simulink model "thermalResistanceNetworkV3"  (R2021b)
settings: Solver=VariableStepAuto  StartTime=0.0  StopTime=numSec  RelTol=1e-3
undefined symbols (not defined in the file): A_rad, A_solararray_face, m_45bracket, m_XRD, Q_PH
libraries: fl_lib x170, nesl_utility x39
(part 1 of 2)
settings Model: Creator=home  LastModifiedBy=benmay

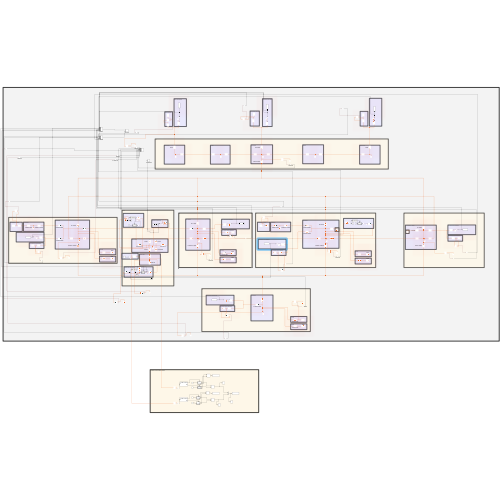
[thumbnail: Simulink's stored preview of the top-level diagram]
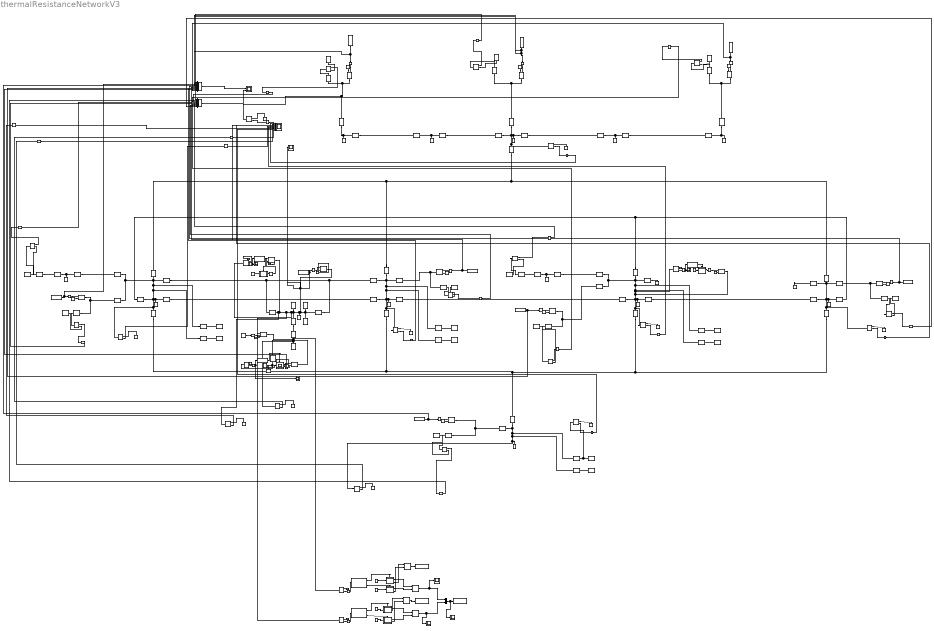
== system thermalResistanceNetworkV3 ==
  note: System
  note: Internal
  note: -X
  note: -Y
  note: Remove
  note: -Z
  note: +Y
  note: +Z Radiator to Space
  note: +Z GRD
  note: +Z XRD
  note: Battery Box
  note: Avioncs Box
  note: +Z Chassis Output Radiation
  note: +Z
  note: +Z Chassis Input Radiation
  note: +X
  note: +Z Radiator
  note: Hinge 2
  note: +X Chassis
  note: Hinge 1
  note: Solar Array 1
  note: Solar Array 2
  note: -X Chassis
  note: +Z Chassis
  note: +Y Chassis
  note: -Y Chassis (To Earth)
  note: -Z Radiator
  note: -Z Chassis
  note: -Z Chassis Output Radiation
  note: -Z Chassis Input Radiation
  note: -X Chassis Output Radiation
  note: -X Chassis Input Radiation
  note: +Y GRD
  note: +Y XRD
  note: -Z GRD
  note: -Z XRD
  note: -X GRD
  note: -X XRD
  note: +Y Chassis Output Radiation
  note: +Y Chassis Input Radiation
  note: -Z Radiator to Space
  note: Remove
  note: -Y Chassis Output Radiation
  note: -Y Chassis Input Radiation
  note: Output Rad SA1
  note: SA1 Input Radiation
  note: +X Chassis Rad Out
  note: +X Chassis Input Rad
  note: Output Rad SA2
  note: SA2 Input Radiation
  note: Battery Heat Gen.
  note: Operational Heat Gen.
  note: Avioncs Box Patch Heater
  note: -Z Patch Heater
  note: Battery Box Patch Heater
  note: PH/RA Brute Force Method Control
  +X Chassis : fl_lib/Thermal/Thermal Elements/Thermal Mass  mass=m_CHX kg  sp_heat=447 J/kg/K  T_specify=off  T_priority=High  T=300 K  T_nominal_specify=off  T_nominal_unit=K  T_nominal_value=1  Q_specify=off  Q_priority=None  Q=0 W  Q_nominal_specify=off  Q_nominal_unit=W  Q_nominal_value=1
  +X Chassis to Hinge 1 : fl_lib/Thermal/Thermal Elements/Thermal Resistance  resistance=R_chassisY K/W  T_specify=off  T_priority=None  T=0 K  T_nominal_specify=off  T_nominal_unit=K  T_nominal_value=1  Q_specify=off  Q_priority=None  Q=0 W  Q_nominal_specify=off  Q_nominal_unit=W  Q_nominal_value=1
      settings: SourceProductBaseCode=SS
  +X Chassis to Hinge 2 : fl_lib/Thermal/Thermal Elements/Thermal Resistance  resistance=R_chassisY K/W  T_specify=off  T_priority=None  T=0 K  T_nominal_specify=off  T_nominal_unit=K  T_nominal_value=1  Q_specify=off  Q_priority=None  Q=0 W  Q_nominal_specify=off  Q_nominal_unit=W  Q_nominal_value=1
      settings: SourceProductBaseCode=SS
  +X Chassis1 : fl_lib/Thermal/Thermal Elements/Thermal Mass  mass=1 kg  sp_heat=447 J/kg/K  T_specify=off  T_priority=High  T=300 K  T_nominal_specify=off  T_nominal_unit=K  T_nominal_value=1  Q_specify=off  Q_priority=None  Q=0 W  Q_nominal_specify=off  Q_nominal_unit=W  Q_nominal_value=1
  +Y Chassis : fl_lib/Thermal/Thermal Elements/Thermal Mass  mass=m_CHYZ kg  sp_heat=447 J/kg/K  T_specify=off  T_priority=High  T=300 K  T_nominal_specify=off  T_nominal_unit=K  T_nominal_value=1  Q_specify=off  Q_priority=None  Q=0 W  Q_nominal_specify=off  Q_nominal_unit=W  Q_nominal_value=1
  +Y Chassis to +Z Chassis : fl_lib/Thermal/Thermal Elements/Thermal Resistance  resistance=R_chassisXZ K/W  T_specify=off  T_priority=None  T=0 K  T_nominal_specify=off  T_nominal_unit=K  T_nominal_value=1  Q_specify=off  Q_priority=None  Q=0 W  Q_nominal_specify=off  Q_nominal_unit=W  Q_nominal_value=1
      settings: SourceProductBaseCode=SS
  +Y Chassis to -X Chassis : fl_lib/Thermal/Thermal Elements/Thermal Resistance  resistance=R_chassisXZ K/W  T_specify=off  T_priority=None  T=0 K  T_nominal_specify=off  T_nominal_unit=K  T_nominal_value=1  Q_specify=off  Q_priority=None  Q=0 W  Q_nominal_specify=off  Q_nominal_unit=W  Q_nominal_value=1
      settings: SourceProductBaseCode=SS
  +Y Chassis to -Z Chassis : fl_lib/Thermal/Thermal Elements/Thermal Resistance  resistance=R_chassisXZ K/W  T_specify=off  T_priority=None  T=0 K  T_nominal_specify=off  T_nominal_unit=K  T_nominal_value=1  Q_specify=off  Q_priority=None  Q=0 W  Q_nominal_specify=off  Q_nominal_unit=W  Q_nominal_value=1
      settings: SourceProductBaseCode=SS
  +Y Chassis to GRD : fl_lib/Thermal/Thermal Elements/Thermal Resistance  resistance=R_XRD K/W  T_specify=off  T_priority=None  T=0 K  T_nominal_specify=off  T_nominal_unit=K  T_nominal_value=1  Q_specify=off  Q_priority=None  Q=0 W  Q_nominal_specify=off  Q_nominal_unit=W  Q_nominal_value=1
      settings: SourceProductBaseCode=SS
  +Y Chassis to Inside : fl_lib/Thermal/Thermal Elements/Thermal Resistance  resistance=R_chassisXZ K/W  T_specify=off  T_priority=None  T=0 K  T_nominal_specify=off  T_nominal_unit=K  T_nominal_value=1  Q_specify=off  Q_priority=None  Q=0 W  Q_nominal_specify=off  Q_nominal_unit=W  Q_nominal_value=1
      settings: SourceProductBaseCode=SS
  +Y Chassis to Outside : fl_lib/Thermal/Thermal Elements/Thermal Resistance  resistance=R_chassisXZ K/W  T_specify=off  T_priority=None  T=0 K  T_nominal_specify=off  T_nominal_unit=K  T_nominal_value=1  Q_specify=off  Q_priority=None  Q=0 W  Q_nominal_specify=off  Q_nominal_unit=W  Q_nominal_value=1
      settings: SourceProductBaseCode=SS
  +Y Chassis to XRD : fl_lib/Thermal/Thermal Elements/Thermal Resistance  resistance=R_XRD K/W  T_specify=off  T_priority=None  T=0 K  T_nominal_specify=off  T_nominal_unit=K  T_nominal_value=1  Q_specify=off  Q_priority=None  Q=0 W  Q_nominal_specify=off  Q_nominal_unit=W  Q_nominal_value=1
      settings: SourceProductBaseCode=SS
  +Y GRD : fl_lib/Thermal/Thermal Elements/Thermal Mass  mass=m_GRD kg  sp_heat=447 J/kg/K  T_specify=off  T_priority=High  T=300 K  T_nominal_specify=off  T_nominal_unit=K  T_nominal_value=1  Q_specify=off  Q_priority=None  Q=0 W  Q_nominal_specify=off  Q_nominal_unit=W  Q_nominal_value=1
  +Y XRD : fl_lib/Thermal/Thermal Elements/Thermal Mass  mass=1.5*m_XRD + 0.5*m_45bracket kg  sp_heat=447 J/kg/K  T_specify=off  T_priority=High  T=300 K  T_nominal_specify=off  T_nominal_unit=K  T_nominal_value=1  Q_specify=off  Q_priority=None  Q=0 W  Q_nominal_specify=off  Q_nominal_unit=W  Q_nominal_value=1
  +Z Chassis : fl_lib/Thermal/Thermal Elements/Thermal Mass  mass=m_CHYZ kg  sp_heat=447 J/kg/K  T_specify=off  T_priority=High  T=300 K  T_nominal_specify=off  T_nominal_unit=K  T_nominal_value=1  Q_specify=off  Q_priority=None  Q=0 W  Q_nominal_specify=off  Q_nominal_unit=W  Q_nominal_value=1
  +Z Chassis to +Y Chassis : fl_lib/Thermal/Thermal Elements/Thermal Resistance  resistance=R_chassisXZ K/W  T_specify=off  T_priority=None  T=0 K  T_nominal_specify=off  T_nominal_unit=K  T_nominal_value=1  Q_specify=off  Q_priority=None  Q=0 W  Q_nominal_specify=off  Q_nominal_unit=W  Q_nominal_value=1
      settings: SourceProductBaseCode=SS
  +Z Chassis to -X Chassis : fl_lib/Thermal/Thermal Elements/Thermal Resistance  resistance=R_chassisXZ K/W  T_specify=off  T_priority=None  T=0 K  T_nominal_specify=off  T_nominal_unit=K  T_nominal_value=1  Q_specify=off  Q_priority=None  Q=0 W  Q_nominal_specify=off  Q_nominal_unit=W  Q_nominal_value=1
      settings: SourceProductBaseCode=SS
  +Z Chassis to -Y Chassis : fl_lib/Thermal/Thermal Elements/Thermal Resistance  resistance=R_chassisXZ K/W  T_specify=off  T_priority=None  T=0 K  T_nominal_specify=off  T_nominal_unit=K  T_nominal_value=1  Q_specify=off  Q_priority=None  Q=0 W  Q_nominal_specify=off  Q_nominal_unit=W  Q_nominal_value=1
      settings: SourceProductBaseCode=SS
  +Z Chassis to GRD : fl_lib/Thermal/Thermal Elements/Thermal Resistance  resistance=R_XRD K/W  T_specify=off  T_priority=None  T=0 K  T_nominal_specify=off  T_nominal_unit=K  T_nominal_value=1  Q_specify=off  Q_priority=None  Q=0 W  Q_nominal_specify=off  Q_nominal_unit=W  Q_nominal_value=1
      settings: SourceProductBaseCode=SS
  +Z Chassis to Inside : fl_lib/Thermal/Thermal Elements/Thermal Resistance  resistance=R_chassisXZ K/W  T_specify=off  T_priority=None  T=0 K  T_nominal_specify=off  T_nominal_unit=K  T_nominal_value=1  Q_specify=off  Q_priority=None  Q=0 W  Q_nominal_specify=off  Q_nominal_unit=W  Q_nominal_value=1
      settings: SourceProductBaseCode=SS
  +Z Chassis to Outside : fl_lib/Thermal/Thermal Elements/Thermal Resistance  resistance=R_chassisXZ K/W  T_specify=off  T_priority=None  T=0 K  T_nominal_specify=off  T_nominal_unit=K  T_nominal_value=1  Q_specify=off  Q_priority=None  Q=0 W  Q_nominal_specify=off  Q_nominal_unit=W  Q_nominal_value=1
      settings: SourceProductBaseCode=SS
  +Z Chassis to Radiator : fl_lib/Thermal/Thermal Elements/Thermal Resistance  resistance=R_chassisXZ K/W  T_specify=off  T_priority=None  T=0 K  T_nominal_specify=off  T_nominal_unit=K  T_nominal_value=1  Q_specify=off  Q_priority=None  Q=0 W  Q_nominal_specify=off  Q_nominal_unit=W  Q_nominal_value=1
      settings: SourceProductBaseCode=SS
  +Z Chassis to XRD : fl_lib/Thermal/Thermal Elements/Thermal Resistance  resistance=R_XRD K/W  T_specify=off  T_priority=None  T=0 K  T_nominal_specify=off  T_nominal_unit=K  T_nominal_value=1  Q_specify=off  Q_priority=None  Q=0 W  Q_nominal_specify=off  Q_nominal_unit=W  Q_nominal_value=1
      settings: SourceProductBaseCode=SS
  +Z GRD : fl_lib/Thermal/Thermal Elements/Thermal Mass  mass=m_GRD kg  sp_heat=447 J/kg/K  T_specify=off  T_priority=High  T=300 K  T_nominal_specify=off  T_nominal_unit=K  T_nominal_value=1  Q_specify=off  Q_priority=None  Q=0 W  Q_nominal_specify=off  Q_nominal_unit=W  Q_nominal_value=1
  +Z Radiator : fl_lib/Thermal/Thermal Elements/Thermal Mass  mass=m_radiator kg  sp_heat=447 J/kg/K  T_specify=off  T_priority=High  T=300 K  T_nominal_specify=off  T_nominal_unit=K  T_nominal_value=1  Q_specify=off  Q_priority=None  Q=0 W  Q_nominal_specify=off  Q_nominal_unit=W  Q_nominal_value=1
  +Z Radiator to +Z Chassis : fl_lib/Thermal/Thermal Elements/Thermal Resistance  resistance=R_rad_chassis_top K/W  T_specify=off  T_priority=None  T=0 K  T_nominal_specify=off  T_nominal_unit=K  T_nominal_value=1  Q_specify=off  Q_priority=None  Q=0 W  Q_nominal_specify=off  Q_nominal_unit=W  Q_nominal_value=1
      settings: SourceProductBaseCode=SS
  +Z Radiator to Space : fl_lib/Thermal/Thermal Elements/Thermal Resistance  resistance=R_rad_chassis_top K/W  T_specify=off  T_priority=None  T=0 K  T_nominal_specify=off  T_nominal_unit=K  T_nominal_value=1  Q_specify=off  Q_priority=None  Q=0 W  Q_nominal_specify=off  Q_nominal_unit=W  Q_nominal_value=1
      settings: SourceProductBaseCode=SS
  +Z XRD : fl_lib/Thermal/Thermal Elements/Thermal Mass  mass=m_XRD kg  sp_heat=447 J/kg/K  T_specify=off  T_priority=High  T=300 K  T_nominal_specify=off  T_nominal_unit=K  T_nominal_value=1  Q_specify=off  Q_priority=None  Q=0 W  Q_nominal_specify=off  Q_nominal_unit=W  Q_nominal_value=1
  -X Chassis to GRD : fl_lib/Thermal/Thermal Elements/Thermal Resistance  resistance=R_XRD K/W  T_specify=off  T_priority=None  T=0 K  T_nominal_specify=off  T_nominal_unit=K  T_nominal_value=1  Q_specify=off  Q_priority=None  Q=0 W  Q_nominal_specify=off  Q_nominal_unit=W  Q_nominal_value=1
      settings: SourceProductBaseCode=SS
  -X Chassis to Outside : fl_lib/Thermal/Thermal Elements/Thermal Resistance  resistance=R_chassisY K/W  T_specify=off  T_priority=None  T=0 K  T_nominal_specify=off  T_nominal_unit=K  T_nominal_value=1  Q_specify=off  Q_priority=None  Q=0 W  Q_nominal_specify=off  Q_nominal_unit=W  Q_nominal_value=1
      settings: SourceProductBaseCode=SS
  -X Chassis to XRD : fl_lib/Thermal/Thermal Elements/Thermal Resistance  resistance=R_XRD K/W  T_specify=off  T_priority=None  T=0 K  T_nominal_specify=off  T_nominal_unit=K  T_nominal_value=1  Q_specify=off  Q_priority=None  Q=0 W  Q_nominal_specify=off  Q_nominal_unit=W  Q_nominal_value=1
      settings: SourceProductBaseCode=SS
  -X GRD : fl_lib/Thermal/Thermal Elements/Thermal Mass  mass=m_GRD kg  sp_heat=447 J/kg/K  T_specify=off  T_priority=High  T=300 K  T_nominal_specify=off  T_nominal_unit=K  T_nominal_value=1  Q_specify=off  Q_priority=None  Q=0 W  Q_nominal_specify=off  Q_nominal_unit=W  Q_nominal_value=1
  -X XRD : fl_lib/Thermal/Thermal Elements/Thermal Mass  mass=1.5*m_XRD + 0.5*m_45bracket kg  sp_heat=447 J/kg/K  T_specify=off  T_priority=High  T=300 K  T_nominal_specify=off  T_nominal_unit=K  T_nominal_value=1  Q_specify=off  Q_priority=None  Q=0 W  Q_nominal_specify=off  Q_nominal_unit=W  Q_nominal_value=1
  -Y Chassis : fl_lib/Thermal/Thermal Elements/Thermal Mass  mass=m_CHYZ kg  sp_heat=447 J/kg/K  T_specify=off  T_priority=High  T=300 K  T_nominal_specify=off  T_nominal_unit=K  T_nominal_value=1  Q_specify=off  Q_priority=None  Q=0 W  Q_nominal_specify=off  Q_nominal_unit=W  Q_nominal_value=1
  -Y Chassis to +Z Chassis : fl_lib/Thermal/Thermal Elements/Thermal Resistance  resistance=R_chassisXZ K/W  T_specify=off  T_priority=None  T=0 K  T_nominal_specify=off  T_nominal_unit=K  T_nominal_value=1  Q_specify=off  Q_priority=None  Q=0 W  Q_nominal_specify=off  Q_nominal_unit=W  Q_nominal_value=1
      settings: SourceProductBaseCode=SS
  -Y Chassis to -Z Chassis : fl_lib/Thermal/Thermal Elements/Thermal Resistance  resistance=R_chassisXZ K/W  T_specify=off  T_priority=None  T=0 K  T_nominal_specify=off  T_nominal_unit=K  T_nominal_value=1  Q_specify=off  Q_priority=None  Q=0 W  Q_nominal_specify=off  Q_nominal_unit=W  Q_nominal_value=1
      settings: SourceProductBaseCode=SS
  -Y to Inside : fl_lib/Thermal/Thermal Elements/Thermal Resistance  resistance=R_chassisXZ K/W  T_specify=off  T_priority=None  T=0 K  T_nominal_specify=off  T_nominal_unit=K  T_nominal_value=1  Q_specify=off  Q_priority=None  Q=0 W  Q_nominal_specify=off  Q_nominal_unit=W  Q_nominal_value=1
      settings: SourceProductBaseCode=SS
  -Y to Outside : fl_lib/Thermal/Thermal Elements/Thermal Resistance  resistance=R_chassisXZ K/W  T_specify=off  T_priority=None  T=0 K  T_nominal_specify=off  T_nominal_unit=K  T_nominal_value=1  Q_specify=off  Q_priority=None  Q=0 W  Q_nominal_specify=off  Q_nominal_unit=W  Q_nominal_value=1
      settings: SourceProductBaseCode=SS
  -Z Chassis : fl_lib/Thermal/Thermal Elements/Thermal Mass  mass=m_CHYZ kg  sp_heat=447 J/kg/K  T_specify=off  T_priority=High  T=300 K  T_nominal_specify=off  T_nominal_unit=K  T_nominal_value=1  Q_specify=off  Q_priority=None  Q=0 W  Q_nominal_specify=off  Q_nominal_unit=W  Q_nominal_value=1
  -Z Chassis to +Y Chassis : fl_lib/Thermal/Thermal Elements/Thermal Resistance  resistance=R_chassisXZ K/W  T_specify=off  T_priority=None  T=0 K  T_nominal_specify=off  T_nominal_unit=K  T_nominal_value=1  Q_specify=off  Q_priority=None  Q=0 W  Q_nominal_specify=off  Q_nominal_unit=W  Q_nominal_value=1
      settings: SourceProductBaseCode=SS
  -Z Chassis to -X Chassis1 : fl_lib/Thermal/Thermal Elements/Thermal Resistance  resistance=R_chassisXZ K/W  T_specify=off  T_priority=None  T=0 K  T_nominal_specify=off  T_nominal_unit=K  T_nominal_value=1  Q_specify=off  Q_priority=None  Q=0 W  Q_nominal_specify=off  Q_nominal_unit=W  Q_nominal_value=1
      settings: SourceProductBaseCode=SS
  -Z Chassis to -Y Chassis : fl_lib/Thermal/Thermal Elements/Thermal Resistance  resistance=R_chassisXZ K/W  T_specify=off  T_priority=None  T=0 K  T_nominal_specify=off  T_nominal_unit=K  T_nominal_value=1  Q_specify=off  Q_priority=None  Q=0 W  Q_nominal_specify=off  Q_nominal_unit=W  Q_nominal_value=1
      settings: SourceProductBaseCode=SS
  -Z Chassis to GRD : fl_lib/Thermal/Thermal Elements/Thermal Resistance  resistance=R_XRD K/W  T_specify=off  T_priority=None  T=0 K  T_nominal_specify=off  T_nominal_unit=K  T_nominal_value=1  Q_specify=off  Q_priority=None  Q=0 W  Q_nominal_specify=off  Q_nominal_unit=W  Q_nominal_value=1
      settings: SourceProductBaseCode=SS
  -Z Chassis to Inside : fl_lib/Thermal/Thermal Elements/Thermal Resistance  resistance=1 K/W  T_specify=off  T_priority=None  T=0 K  T_nominal_specify=off  T_nominal_unit=K  T_nominal_value=1  Q_specify=off  Q_priority=None  Q=0 W  Q_nominal_specify=off  Q_nominal_unit=W  Q_nominal_value=1
      settings: SourceProductBaseCode=SS
  -Z Chassis to Outside : fl_lib/Thermal/Thermal Elements/Thermal Resistance  resistance=R_chassisXZ K/W  T_specify=off  T_priority=None  T=0 K  T_nominal_specify=off  T_nominal_unit=K  T_nominal_value=1  Q_specify=off  Q_priority=None  Q=0 W  Q_nominal_specify=off  Q_nominal_unit=W  Q_nominal_value=1
      settings: SourceProductBaseCode=SS
  -Z Chassis to Radiator : fl_lib/Thermal/Thermal Elements/Thermal Resistance  resistance=R_chassisXZ K/W  T_specify=off  T_priority=None  T=0 K  T_nominal_specify=off  T_nominal_unit=K  T_nominal_value=1  Q_specify=off  Q_priority=None  Q=0 W  Q_nominal_specify=off  Q_nominal_unit=W  Q_nominal_value=1
      settings: SourceProductBaseCode=SS
  -Z Chassis to XRD : fl_lib/Thermal/Thermal Elements/Thermal Resistance  resistance=R_XRD K/W  T_specify=off  T_priority=None  T=0 K  T_nominal_specify=off  T_nominal_unit=K  T_nominal_value=1  Q_specify=off  Q_priority=None  Q=0 W  Q_nominal_specify=off  Q_nominal_unit=W  Q_nominal_value=1
      settings: SourceProductBaseCode=SS
  -Z GRD : fl_lib/Thermal/Thermal Elements/Thermal Mass  mass=m_GRD kg  sp_heat=447 J/kg/K  T_specify=off  T_priority=High  T=300 K  T_nominal_specify=off  T_nominal_unit=K  T_nominal_value=1  Q_specify=off  Q_priority=None  Q=0 W  Q_nominal_specify=off  Q_nominal_unit=W  Q_nominal_value=1
  -Z Radiator : fl_lib/Thermal/Thermal Elements/Thermal Mass  mass=m_radiator kg  sp_heat=447 J/kg/K  T_specify=off  T_priority=High  T=300 K  T_nominal_specify=off  T_nominal_unit=K  T_nominal_value=1  Q_specify=off  Q_priority=None  Q=0 W  Q_nominal_specify=off  Q_nominal_unit=W  Q_nominal_value=1
  -Z Radiator to -Z Chassis : fl_lib/Thermal/Thermal Elements/Thermal Resistance  resistance=R_chassisXZ K/W  T_specify=off  T_priority=None  T=0 K  T_nominal_specify=off  T_nominal_unit=K  T_nominal_value=1  Q_specify=off  Q_priority=None  Q=0 W  Q_nominal_specify=off  Q_nominal_unit=W  Q_nominal_value=1
      settings: SourceProductBaseCode=SS
  -Z Radiator to Space : fl_lib/Thermal/Thermal Elements/Thermal Resistance  resistance=R_chassisXZ K/W  T_specify=off  T_priority=None  T=0 K  T_nominal_specify=off  T_nominal_unit=K  T_nominal_value=1  Q_specify=off  Q_priority=None  Q=0 W  Q_nominal_specify=off  Q_nominal_unit=W  Q_nominal_value=1
      settings: SourceProductBaseCode=SS
  -Z XRD : fl_lib/Thermal/Thermal Elements/Thermal Mass  mass=2*m_XRD + 0.5*m_45bracket kg  sp_heat=447 J/kg/K  T_specify=off  T_priority=High  T=300 K  T_nominal_specify=off  T_nominal_unit=K  T_nominal_value=1  Q_specify=off  Q_priority=None  Q=0 W  Q_nominal_specify=off  Q_nominal_unit=W  Q_nominal_value=1
  Avionics -Y : fl_lib/Thermal/Thermal Elements/Thermal Resistance  resistance=R_AB_internal K/W  T_specify=off  T_priority=None  T=0 K  T_nominal_specify=off  T_nominal_unit=K  T_nominal_value=1  Q_specify=off  Q_priority=None  Q=0 W  Q_nominal_specify=off  Q_nominal_unit=W  Q_nominal_value=1
      settings: SourceProductBaseCode=SS
  Avionics -Z : fl_lib/Thermal/Thermal Elements/Thermal Resistance  resistance=1 K/W  T_specify=off  T_priority=None  T=0 K  T_nominal_specify=off  T_nominal_unit=K  T_nominal_value=1  Q_specify=off  Q_priority=None  Q=0 W  Q_nominal_specify=off  Q_nominal_unit=W  Q_nominal_value=1
      settings: SourceProductBaseCode=SS
  Avionics Bottom : fl_lib/Thermal/Thermal Elements/Thermal Resistance  resistance=1 K/W  T_specify=off  T_priority=None  T=0 K  T_nominal_specify=off  T_nominal_unit=K  T_nominal_value=1  Q_specify=off  Q_priority=None  Q=0 W  Q_nominal_specify=off  Q_nominal_unit=W  Q_nominal_value=1
      settings: SourceProductBaseCode=SS
  Avionics Box : fl_lib/Thermal/Thermal Elements/Thermal Mass  mass=m_AB kg  sp_heat=447 J/kg/K  T_specify=on  T_priority=High  T=282 K  T_nominal_specify=off  T_nominal_unit=K  T_nominal_value=1  Q_specify=off  Q_priority=None  Q=0 W  Q_nominal_specify=off  Q_nominal_unit=W  Q_nominal_value=1
  Avionics Box to +Y : fl_lib/Thermal/Thermal Elements/Thermal Resistance  resistance=R_AB_internal K/W  T_specify=off  T_priority=None  T=0 K  T_nominal_specify=off  T_nominal_unit=K  T_nominal_value=1  Q_specify=off  Q_priority=None  Q=0 W  Q_nominal_specify=off  Q_nominal_unit=W  Q_nominal_value=1
      settings: SourceProductBaseCode=SS
  Avionics Box to +Z : fl_lib/Thermal/Thermal Elements/Thermal Resistance  resistance=R_AB_internal K/W  T_specify=off  T_priority=None  T=0 K  T_nominal_specify=off  T_nominal_unit=K  T_nominal_value=1  Q_specify=off  Q_priority=None  Q=0 W  Q_nominal_specify=off  Q_nominal_unit=W  Q_nominal_value=1
      settings: SourceProductBaseCode=SS
  Avionics Top : fl_lib/Thermal/Thermal Elements/Thermal Resistance  resistance=1 K/W  T_specify=off  T_priority=None  T=0 K  T_nominal_specify=off  T_nominal_unit=K  T_nominal_value=1  Q_specify=off  Q_priority=None  Q=0 W  Q_nominal_specify=off  Q_nominal_unit=W  Q_nominal_value=1
      settings: SourceProductBaseCode=SS
  AvionicsBox : nesl_utility/PS-Simulink Converter  PhysicalDomain=network_engine_domain  SubClassName=ps_output  LeftPortType=input  RightPortType=output  PseudoPeriodic=off  Frequencies=[]  Unit=K  AffineConversion=off
      settings: SourceProductBaseCode=PW,SS
  Battery Box : fl_lib/Thermal/Thermal Elements/Thermal Mass  mass=m_BB kg  sp_heat=447 J/kg/K  T_specify=on  T_priority=High  T=282 K  T_nominal_specify=off  T_nominal_unit=K  T_nominal_value=1  Q_specify=off  Q_priority=None  Q=0 W  Q_nominal_specify=off  Q_nominal_unit=W  Q_nominal_value=1
  Battery Box to Avionics : fl_lib/Thermal/Thermal Elements/Thermal Resistance  resistance=R_BB_internal K/W  T_specify=off  T_priority=None  T=0 K  T_nominal_specify=off  T_nominal_unit=K  T_nominal_value=1  Q_specify=off  Q_priority=None  Q=0 W  Q_nominal_specify=off  Q_nominal_unit=W  Q_nominal_value=1
      settings: SourceProductBaseCode=SS
  BatteryBox : nesl_utility/PS-Simulink Converter  PhysicalDomain=network_engine_domain  SubClassName=ps_output  LeftPortType=input  RightPortType=output  PseudoPeriodic=off  Frequencies=[]  Unit=K  AffineConversion=off
      settings: SourceProductBaseCode=PW,SS
  "Bottom +X Chassis " : fl_lib/Thermal/Thermal Elements/Thermal Resistance  resistance=R_chassisY K/W  T_specify=off  T_priority=None  T=0 K  T_nominal_specify=off  T_nominal_unit=K  T_nominal_value=1  Q_specify=off  Q_priority=None  Q=0 W  Q_nominal_specify=off  Q_nominal_unit=W  Q_nominal_value=1
      settings: SourceProductBaseCode=SS
  "Bottom -Y Chassis " : fl_lib/Thermal/Thermal Elements/Thermal Resistance  resistance=R_chassisXZ K/W  T_specify=off  T_priority=None  T=0 K  T_nominal_specify=off  T_nominal_unit=K  T_nominal_value=1  Q_specify=off  Q_priority=None  Q=0 W  Q_nominal_specify=off  Q_nominal_unit=W  Q_nominal_value=1
      settings: SourceProductBaseCode=SS
  Constant : Constant  Value=0.9
  Constant1 : Constant  Value=0
  Constant2 : Constant  Value=Q_PH/3
  Constant3 : Constant  Value=0
  Constant4 : Constant
  Constant5 : Constant
  Constant6 : Constant  Value=Q_PH/3
  Constant7 : Constant  Value=Q_PH/3
  Controlled Heat Flow Rate Source{,1..12} (13 alike) : fl_lib/Thermal/Thermal Sources/Controlled Heat Flow Rate Source
  From Workspace1 : FromWorkspace  VariableName=Q_SA_TS  SampleTime=300
  From Workspace10 : FromWorkspace  VariableName=Q_Gen_TS  SampleTime=300
  From Workspace2 : FromWorkspace  VariableName=Q_Xpos_TS  SampleTime=300
  From Workspace3 : FromWorkspace  VariableName=Q_SA_TS  SampleTime=300
  From Workspace4 : FromWorkspace  VariableName=Q_Zpos_TS  SampleTime=300
  From Workspace5 : FromWorkspace  VariableName=Q_Ypos_TS  SampleTime=300
  From Workspace6 : FromWorkspace  VariableName=Q_Zneg_TS  SampleTime=300
  From Workspace7 : FromWorkspace  VariableName=Q_Xneg_TS  SampleTime=300
  From Workspace8 : FromWorkspace  VariableName=Q_Yneg_TS  SampleTime=300
  Heat Flow Rate Sensor{1..10} (10 alike) : fl_lib/Thermal/Thermal Sensors/Heat Flow Rate Sensor
      settings: SourceProductBaseCode=SS
  Heat In : Sum  Inputs=+++++++++++
  Heat Out : Sum  Inputs=++++++++++
  Heat in/out : Scope  NumInputPorts=2
  Hinge 1 : fl_lib/Thermal/Thermal Elements/Thermal Mass  mass=m_hinge kg  sp_heat=887 J/kg/K  T_specify=off  T_priority=High  T=300 K  T_nominal_specify=off  T_nominal_unit=K  T_nominal_value=1  Q_specify=off  Q_priority=None  Q=0 W  Q_nominal_specify=off  Q_nominal_unit=W  Q_nominal_value=1
  Hinge 1 to +X Chassis : fl_lib/Thermal/Thermal Elements/Thermal Resistance  resistance=R_Hinge K/W  T_specify=off  T_priority=None  T=0 K  T_nominal_specify=off  T_nominal_unit=K  T_nominal_value=1  Q_specify=off  Q_priority=None  Q=0 W  Q_nominal_specify=off  Q_nominal_unit=W  Q_nominal_value=1
      settings: SourceProductBaseCode=SS
  Hinge 1 to SA1 : fl_lib/Thermal/Thermal Elements/Thermal Resistance  resistance=R_Hinge K/W  T_specify=off  T_priority=None  T=0 K  T_nominal_specify=off  T_nominal_unit=K  T_nominal_value=1  Q_specify=off  Q_priority=None  Q=0 W  Q_nominal_specify=off  Q_nominal_unit=W  Q_nominal_value=1
      settings: SourceProductBaseCode=SS
  Hinge 2 : fl_lib/Thermal/Thermal Elements/Thermal Mass  mass=m_hinge kg  sp_heat=447 J/kg/K  T_specify=off  T_priority=High  T=300 K  T_nominal_specify=off  T_nominal_unit=K  T_nominal_value=1  Q_specify=off  Q_priority=None  Q=0 W  Q_nominal_specify=off  Q_nominal_unit=W  Q_nominal_value=1
  Hinge 2 to +X Chassis : fl_lib/Thermal/Thermal Elements/Thermal Resistance  resistance=R_Hinge K/W  T_specify=off  T_priority=None  T=0 K  T_nominal_specify=off  T_nominal_unit=K  T_nominal_value=1  Q_specify=off  Q_priority=None  Q=0 W  Q_nominal_specify=off  Q_nominal_unit=W  Q_nominal_value=1
      settings: SourceProductBaseCode=SS
  Hinge 2 to SA2 : fl_lib/Thermal/Thermal Elements/Thermal Resistance  resistance=R_Hinge K/W  T_specify=off  T_priority=None  T=0 K  T_nominal_specify=off  T_nominal_unit=K  T_nominal_value=1  Q_specify=off  Q_priority=None  Q=0 W  Q_nominal_specify=off  Q_nominal_unit=W  Q_nominal_value=1
      settings: SourceProductBaseCode=SS
  If Action Subsystem1 : Subsystem  TreatAsAtomicUnit=on
  If Action Subsystem2 : Subsystem  TreatAsAtomicUnit=on
  If Action Subsystem3 : Subsystem  TreatAsAtomicUnit=on
  If Action Subsystem4 : Subsystem  TreatAsAtomicUnit=on
  If Action Subsystem5 : Subsystem  TreatAsAtomicUnit=on
  If Action Subsystem6 : Subsystem  TreatAsAtomicUnit=on
  If Action Subsystem7 : Subsystem  TreatAsAtomicUnit=on
  If1 : If  IfExpression=u1 > 288.5 | u1<278.15
  If2 : If  IfExpression=u1 < 283.15  ShowElse=off
  If3 : If  IfExpression=u1 < 273.15  ShowElse=off
  If4 : If  IfExpression=u1 > 308.5 | u1<278.15
  If5 : If  IfExpression=u1 < 288.15  ShowElse=off
  Inside Edge SA1 : fl_lib/Thermal/Thermal Elements/Thermal Resistance  resistance=R_SolarArray K/W  T_specify=off  T_priority=None  T=0 K  T_nominal_specify=off  T_nominal_unit=K  T_nominal_value=1  Q_specify=off  Q_priority=None  Q=0 W  Q_nominal_specify=off  Q_nominal_unit=W  Q_nominal_value=1
      settings: SourceProductBaseCode=SS
  Merge{,1..3} (4 alike) : Merge
  Mux : Mux  Inputs=2
  Outside Edge SA2 : fl_lib/Thermal/Thermal Elements/Thermal Resistance  resistance=R_SolarArray K/W  T_specify=off  T_priority=None  T=0 K  T_nominal_specify=off  T_nominal_unit=K  T_nominal_value=1  Q_specify=off  Q_priority=None  Q=0 W  Q_nominal_specify=off  Q_nominal_unit=W  Q_nominal_value=1
      settings: SourceProductBaseCode=SS
  PS-Simulink Converter{1..15} (15 alike) : nesl_utility/PS-Simulink Converter  PhysicalDomain=network_engine_domain  SubClassName=ps_output  LeftPortType=input  RightPortType=output  PseudoPeriodic=off  Frequencies=[]  Unit=inherit  AffineConversion=off
      settings: SourceProductBaseCode=PW,SS
  Perfect Insulator : fl_lib/Thermal/Thermal Elements/Perfect Insulator  T_specify=off  T_priority=None  T=0 K  T_nominal_specify=off  T_nominal_unit=K  T_nominal_value=1
  Perfect Insulator1 : fl_lib/Thermal/Thermal Elements/Perfect Insulator  T_specify=off  T_priority=None  T=0 K  T_nominal_specify=off  T_nominal_unit=K  T_nominal_value=1
  Power Generated : Scope
  Radiative Heat Transfer{,1,4,6} (4 alike) : fl_lib/Thermal/Thermal Elements/Radiative Heat Transfer  area=A_sidechassis m^2  rad_tr_coeff=RC_Al W/(m^2*K^4)  T_specify=off  T_priority=None  T=0 K  T_nominal_specify=off  T_nominal_unit=K  T_nominal_value=1  Q_specify=off  Q_priority=None  Q=0 W  Q_nominal_specify=off  Q_nominal_unit=W  Q_nominal_value=1
      settings: SourceProductBaseCode=SS  InternalSimscapePortConfiguration="{\"Bottom\":[],\"Left\":[{\"id\":\"A\",\"label\":\"A\",\"type\":\"foundation.thermal.thermal\"}],\"Right\":[{\"id\":\"B\",\"label\":\"B\",\"type\":\"foundation.thermal.thermal\"}],\"Top\":[]}"
  Radiative Heat Transfer2 : fl_lib/Thermal/Thermal Elements/Radiative Heat Transfer  area=A_topchassis m^2  rad_tr_coeff=RC_Al W/(m^2*K^4)  T_specify=off  T_priority=None  T=0 K  T_nominal_specify=off  T_nominal_unit=K  T_nominal_value=1  Q_specify=off  Q_priority=None  Q=0 W  Q_nominal_specify=off  Q_nominal_unit=W  Q_nominal_value=1
      settings: SourceProductBaseCode=SS  InternalSimscapePortConfiguration="{\"Bottom\":[],\"Left\":[{\"id\":\"A\",\"label\":\"A\",\"type\":\"foundation.thermal.thermal\"}],\"Right\":[{\"id\":\"B\",\"label\":\"B\",\"type\":\"foundation.thermal.thermal\"}],\"Top\":[]}"
  Radiative Heat Transfer3 : fl_lib/Thermal/Thermal Elements/Radiative Heat Transfer  area=A_rad/2 m^2  rad_tr_coeff=RC_Rad W/(m^2*K^4)  T_specify=off  T_priority=None  T=0 K  T_nominal_specify=off  T_nominal_unit=K  T_nominal_value=1  Q_specify=off  Q_priority=None  Q=0 W  Q_nominal_specify=off  Q_nominal_unit=W  Q_nominal_value=1
      settings: SourceProductBaseCode=SS  InternalSimscapePortConfiguration="{\"Bottom\":[],\"Left\":[{\"id\":\"A\",\"label\":\"A\",\"type\":\"foundation.thermal.thermal\"}],\"Right\":[{\"id\":\"B\",\"label\":\"B\",\"type\":\"foundation.thermal.thermal\"}],\"Top\":[]}"
  Radiative Heat Transfer5 : fl_lib/Thermal/Thermal Elements/Radiative Heat Transfer  area=A_rad/2 m^2  rad_tr_coeff=RC_Rad W/(m^2*K^4)  T_specify=off  T_priority=None  T=0 K  T_nominal_specify=off  T_nominal_unit=K  T_nominal_value=1  Q_specify=off  Q_priority=None  Q=0 W  Q_nominal_specify=off  Q_nominal_unit=W  Q_nominal_value=1
      settings: SourceProductBaseCode=SS  InternalSimscapePortConfiguration="{\"Bottom\":[],\"Left\":[{\"id\":\"A\",\"label\":\"A\",\"type\":\"foundation.thermal.thermal\"}],\"Right\":[{\"id\":\"B\",\"label\":\"B\",\"type\":\"foundation.thermal.thermal\"}],\"Top\":[]}"
  Radiative Heat Transfer7 : fl_lib/Thermal/Thermal Elements/Radiative Heat Transfer  area=2*A_solararray_face m^2  rad_tr_coeff=RC_SA W/(m^2*K^4)  T_specify=off  T_priority=None  T=0 K  T_nominal_specify=off  T_nominal_unit=K  T_nominal_value=1  Q_specify=off  Q_priority=None  Q=0 W  Q_nominal_specify=off  Q_nominal_unit=W  Q_nominal_value=1
      settings: SourceProductBaseCode=SS  InternalSimscapePortConfiguration="{\"Bottom\":[],\"Left\":[{\"id\":\"A\",\"label\":\"A\",\"type\":\"foundation.thermal.thermal\"}],\"Right\":[{\"id\":\"B\",\"label\":\"B\",\"type\":\"foundation.thermal.thermal\"}],\"Top\":[]}"
  Radiative Heat Transfer8 : fl_lib/Thermal/Thermal Elements/Radiative Heat Transfer  area=A_topchassis m^2  rad_tr_coeff=RC_Al W/(m^2*K^4)  T_specify=off  T_priority=None  T=0 K  T_nominal_specify=off  T_nominal_unit=K  T_nominal_value=1  Q_specify=off  Q_priority=None  Q=0 W  Q_nominal_specify=off  Q_nominal_unit=W  Q_nominal_value=1
      settings: SourceProductBaseCode=SS  InternalSimscapePortConfiguration="{\"Bottom\":[],\"Left\":[{\"id\":\"A\",\"label\":\"A\",\"type\":\"foundation.thermal.thermal\"}],\"Right\":[{\"id\":\"B\",\"label\":\"B\",\"type\":\"foundation.thermal.thermal\"}],\"Top\":[]}"
  Radiative Heat Transfer9 : fl_lib/Thermal/Thermal Elements/Radiative Heat Transfer  area=2*A_solararray_face m^2  rad_tr_coeff=RC_SA W/(m^2*K^4)  T_specify=off  T_priority=None  T=0 K  T_nominal_specify=off  T_nominal_unit=K  T_nominal_value=1  Q_specify=off  Q_priority=None  Q=0 W  Q_nominal_specify=off  Q_nominal_unit=W  Q_nominal_value=1
      settings: SourceProductBaseCode=SS  InternalSimscapePortConfiguration="{\"Bottom\":[],\"Left\":[{\"id\":\"A\",\"label\":\"A\",\"type\":\"foundation.thermal.thermal\"}],\"Right\":[{\"id\":\"B\",\"label\":\"B\",\"type\":\"foundation.thermal.thermal\"}],\"Top\":[]}"
  SA1 : fl_lib/Thermal/Thermal Elements/Thermal Mass  mass=m_SA kg  sp_heat=887 J/kg/K  T_specify=off  T_priority=High  T=300 K  T_nominal_specify=off  T_nominal_unit=K  T_nominal_value=1  Q_specify=off  Q_priority=None  Q=0 W  Q_nominal_specify=off  Q_nominal_unit=W  Q_nominal_value=1
  SA2 : fl_lib/Thermal/Thermal Elements/Thermal Mass  mass=m_SA kg  sp_heat=887 J/kg/K  T_specify=off  T_priority=High  T=300 K  T_nominal_specify=off  T_nominal_unit=K  T_nominal_value=1  Q_specify=off  Q_priority=None  Q=0 W  Q_nominal_specify=off  Q_nominal_unit=W  Q_nominal_value=1
  Scope{,1..5} (6 alike) : Scope
  Simulink-PS Converter{,1..12} (13 alike) : nesl_utility/Simulink-PS Converter  PhysicalDomain=network_engine_domain  SubClassName=ps_input  LeftPortType=input  RightPortType=output  PseudoPeriodic=off  Frequencies=[]  NoiseDistribution=none  NoiseParameters=[]  Unit=1  AffineConversion=off  FilteringAndDerivatives=provide  SimscapeFilterOrder=1  InputFilterTimeConstant=0.001  UdotUserProvided=0
      settings: SourceProductBaseCode=PW,SS
  Solar Array : nesl_utility/PS-Simulink Converter  PhysicalDomain=network_engine_domain  SubClassName=ps_output  LeftPortType=input  RightPortType=output  PseudoPeriodic=off  Frequencies=[]  Unit=K  AffineConversion=off
      settings: SourceProductBaseCode=PW,SS
  Solver Configuration : nesl_utility/Solver Configuration  PhysicalDomain=network_engine_domain  SubClassName=solver  LeftPortType=input  RightPortType=generic  Tones=[]  Harmonics=[]  SimulateNoise=off  Profile=off  UseLocalSampling=off  EnableSwitchedLinearOptims=on  FrequencyDomain=off  UseCCode=off  RelTol=0.001  AbsTol=1e-06  MinStep=1e-09  ToWorkspace=off  RevertToSquareIcSolve=off  NumHomotopyIterations=100  PhasorMode=off  PhasorModeNumHarmonics=1  DoDC=off  ResidualTolerance=1e-09  UseLocalSolver=off  LocalSolverChoice=NE_BACKWARD_EULER_ADVANCER  LocalSolverSampleTime=0.001  DoFixedCost=off  MaxNonlinIter=3  MaxModeIter=2  ComputeImpulses=off  ImpulseIterations=2  LinearAlgebra=auto  EquationFormulation=NE_TIME_EF  DelaysMemoryBudget=1024  AutomaticFiltering=on  FilteringTimeConstant=0.001  PartitionStorageMethod=AS_NEEDED  PartitionMemoryBudget=1024  PartitionMethod=ROBUST
      settings: SourceProductBaseCode=PW,SS
  Space{,1..9} (10 alike) : fl_lib/Thermal/Thermal Sources/Temperature Source  temperature=2.7 K
  Temperature Sensor{1..15} (15 alike) : fl_lib/Thermal/Thermal Sensors/Temperature Sensor
  Temperatures : Scope  NumInputPorts=10
  Thermal Reference{,1..27} (28 alike) : fl_lib/Thermal/Thermal Elements/Thermal Reference
  Thermal Resistance : fl_lib/Thermal/Thermal Elements/Thermal Resistance  resistance=1 K/W  T_specify=off  T_priority=None  T=0 K  T_nominal_specify=off  T_nominal_unit=K  T_nominal_value=1  Q_specify=off  Q_priority=None  Q=0 W  Q_nominal_specify=off  Q_nominal_unit=W  Q_nominal_value=1
      settings: SourceProductBaseCode=SS
  To Workspace : ToWorkspace  VariableName=BB_Results  SampleTime=300
  To Workspace1 : ToWorkspace  VariableName=Avionics_Results  SampleTime=300
  To Workspace2 : ToWorkspace  VariableName=Combined_Results  SampleTime=300
  "Top +X Chassis " : fl_lib/Thermal/Thermal Elements/Thermal Resistance  resistance=R_chassisY K/W  T_specify=off  T_priority=None  T=0 K  T_nominal_specify=off  T_nominal_unit=K  T_nominal_value=1  Q_specify=off  Q_priority=None  Q=0 W  Q_nominal_specify=off  Q_nominal_unit=W  Q_nominal_value=1
      settings: SourceProductBaseCode=SS
  Top +Y Chassis : fl_lib/Thermal/Thermal Elements/Thermal Resistance  resistance=R_chassisXZ K/W  T_specify=off  T_priority=None  T=0 K  T_nominal_specify=off  T_nominal_unit=K  T_nominal_value=1  Q_specify=off  Q_priority=None  Q=0 W  Q_nominal_specify=off  Q_nominal_unit=W  Q_nominal_value=1
      settings: SourceProductBaseCode=SS
  Top +Z Chassis : fl_lib/Thermal/Thermal Elements/Thermal Resistance  resistance=R_chassisXZ K/W  T_specify=off  T_priority=None  T=0 K  T_nominal_specify=off  T_nominal_unit=K  T_nominal_value=1  Q_specify=off  Q_priority=None  Q=0 W  Q_nominal_specify=off  Q_nominal_unit=W  Q_nominal_value=1
      settings: SourceProductBaseCode=SS
  Top -X Chassis : fl_lib/Thermal/Thermal Elements/Thermal Resistance  resistance=R_chassisY K/W  T_specify=off  T_priority=None  T=0 K  T_nominal_specify=off  T_nominal_unit=K  T_nominal_value=1  Q_specify=off  Q_priority=None  Q=0 W  Q_nominal_specify=off  Q_nominal_unit=W  Q_nominal_value=1
      settings: SourceProductBaseCode=SS
  "Top -Y Chassis " : fl_lib/Thermal/Thermal Elements/Thermal Resistance  resistance=R_chassisXZ K/W  T_specify=off  T_priority=None  T=0 K  T_nominal_specify=off  T_nominal_unit=K  T_nominal_value=1  Q_specify=off  Q_priority=None  Q=0 W  Q_nominal_specify=off  Q_nominal_unit=W  Q_nominal_value=1
      settings: SourceProductBaseCode=SS
  Top -Z Chassis : fl_lib/Thermal/Thermal Elements/Thermal Resistance  resistance=R_chassisXZ K/W  T_specify=off  T_priority=None  T=0 K  T_nominal_specify=off  T_nominal_unit=K  T_nominal_value=1  Q_specify=off  Q_priority=None  Q=0 W  Q_nominal_specify=off  Q_nominal_unit=W  Q_nominal_value=1
      settings: SourceProductBaseCode=SS
  Top SA1 : fl_lib/Thermal/Thermal Elements/Thermal Resistance  resistance=R_SolarArray K/W  T_specify=off  T_priority=None  T=0 K  T_nominal_specify=off  T_nominal_unit=K  T_nominal_value=1  Q_specify=off  Q_priority=None  Q=0 W  Q_nominal_specify=off  Q_nominal_unit=W  Q_nominal_value=1
      settings: SourceProductBaseCode=SS
  Top SA2 : fl_lib/Thermal/Thermal Elements/Thermal Resistance  resistance=R_SolarArray K/W  T_specify=off  T_priority=None  T=0 K  T_nominal_specify=off  T_nominal_unit=K  T_nominal_value=1  Q_specify=off  Q_priority=None  Q=0 W  Q_nominal_specify=off  Q_nominal_unit=W  Q_nominal_value=1
      settings: SourceProductBaseCode=SS
  X+ chassis face : nesl_utility/PS-Simulink Converter  PhysicalDomain=network_engine_domain  SubClassName=ps_output  LeftPortType=input  RightPortType=output  PseudoPeriodic=off  Frequencies=[]  Unit=K  AffineConversion=off
      settings: SourceProductBaseCode=PW,SS
  X- chassis face : nesl_utility/PS-Simulink Converter  PhysicalDomain=network_engine_domain  SubClassName=ps_output  LeftPortType=input  RightPortType=output  PseudoPeriodic=off  Frequencies=[]  Unit=K  AffineConversion=off
      settings: SourceProductBaseCode=PW,SS
  XRD (X-) : nesl_utility/PS-Simulink Converter  PhysicalDomain=network_engine_domain  SubClassName=ps_output  LeftPortType=input  RightPortType=output  PseudoPeriodic=off  Frequencies=[]  Unit=K  AffineConversion=off
      settings: SourceProductBaseCode=PW,SS
  Y+ chassis face : nesl_utility/PS-Simulink Converter  PhysicalDomain=network_engine_domain  SubClassName=ps_output  LeftPortType=input  RightPortType=output  PseudoPeriodic=off  Frequencies=[]  Unit=K  AffineConversion=off
      settings: SourceProductBaseCode=PW,SS
  Y- chassis face : nesl_utility/PS-Simulink Converter  PhysicalDomain=network_engine_domain  SubClassName=ps_output  LeftPortType=input  RightPortType=output  PseudoPeriodic=off  Frequencies=[]  Unit=K  AffineConversion=off
      settings: SourceProductBaseCode=PW,SS
  Z+ chassis Face : nesl_utility/PS-Simulink Converter  PhysicalDomain=network_engine_domain  SubClassName=ps_output  LeftPortType=input  RightPortType=output  PseudoPeriodic=off  Frequencies=[]  Unit=K  AffineConversion=off
      settings: SourceProductBaseCode=PW,SS
  Z- chassis face : nesl_utility/PS-Simulink Converter  PhysicalDomain=network_engine_domain  SubClassName=ps_output  LeftPortType=input  RightPortType=output  PseudoPeriodic=off  Frequencies=[]  Unit=K  AffineConversion=off
      settings: SourceProductBaseCode=PW,SS
  wires:
  Solar Array/1 -> Temperatures/7
  BatteryBox/1 -> Temperatures/10
  AvionicsBox/1 -> Temperatures/8
  X- chassis face/1 -> Temperatures/2
  Heat In/1 -> Heat in/out/1
  From Workspace2/1 -> Heat In/5, Heat In/2, Simulink-PS Converter6/1
  From Workspace4/1 -> Heat In/3, Simulink-PS Converter/1
  From Workspace7/1 -> Heat In/4, Simulink-PS Converter2/1
  From Workspace8/1 -> Heat In/6, Simulink-PS Converter4/1
  From Workspace5/1 -> Heat In/7, Simulink-PS Converter3/1
  From Workspace6/1 -> Simulink-PS Converter1/1, Heat In/8
  Heat Out/1 -> Heat in/out/2
  PS-Simulink Converter2/1 -> Heat Out/1
  PS-Simulink Converter3/1 -> Heat Out/4
  PS-Simulink Converter4/1 -> Heat Out/5
  PS-Simulink Converter5/1 -> Heat Out/6
  PS-Simulink Converter6/1 -> Heat Out/3
  PS-Simulink Converter7/1 -> Heat Out/7
  PS-Simulink Converter8/1 -> Heat Out/8
  PS-Simulink Converter9/1 -> Heat Out/9
  PS-Simulink Converter10/1 -> Heat Out/10
  Constant2/1 -> If Action Subsystem2/1(In1)
  PS-Simulink Converter11/1 -> If2/1, Scope3/1
  If Action Subsystem2/1(Out1) -> Simulink-PS Converter9/1
  If2/1 -> If Action Subsystem2/Action
  From Workspace1/1 -> Heat In/1, Simulink-PS Converter5/1
  PS-Simulink Converter12/1 -> Heat Out/2
  Constant/1 -> Simulink-PS Converter8/1
  From Workspace10/1 -> Simulink-PS Converter10/1, Power Generated/1, Heat In/9
  Z+ chassis Face/1 -> Temperatures/5
  X+ chassis face/1 -> Temperatures/1
  Y- chassis face/1 -> Temperatures/4
  Z- chassis face/1 -> Temperatures/6
  Y+ chassis face/1 -> Temperatures/3
  XRD (X-)/1 -> Temperatures/9
  If Action Subsystem2/2(Out2) -> Heat In/10
  From Workspace3/1 -> Heat In/11, Simulink-PS Converter7/1
  PS-Simulink Converter1/1 -> If1/1
  Constant1/1 -> If Action Subsystem1/1(In1)
  If1/1 -> If Action Subsystem1/Action
  If4/1 -> If Action Subsystem3/Action
  Constant3/1 -> If Action Subsystem3/1(In1)
  PS-Simulink Converter13/1 -> If4/1
  Constant4/1 -> If Action Subsystem4/1(In1)
  If4/2 -> If Action Subsystem4/Action
  Constant5/1 -> If Action Subsystem5/1(In1)
  If1/2 -> If Action Subsystem5/Action
  If Action Subsystem4/1(Out1) -> Merge2/2
  If Action Subsystem3/1(Out1) -> Merge2/1
  If Action Subsystem1/1(Out1) -> Merge/1
  If Action Subsystem5/1(Out1) -> Merge/2
  Merge/1 -> Scope2/1, Mux/1
  If Action Subsystem1/2(Out2) -> Merge1/1
  If Action Subsystem5/2(Out2) -> Merge1/2
  Merge1/1 -> To Workspace/1
  If Action Subsystem3/2(Out2) -> Merge3/1
  If Action Subsystem4/2(Out2) -> Merge3/2
  Merge3/1 -> To Workspace1/1
  Merge2/1 -> Scope/1, Mux/2
  Mux/1 -> Scope1/1, To Workspace2/1
  If3/1 -> If Action Subsystem6/Action
  If Action Subsystem6/1(Out1) -> Simulink-PS Converter11/1
  PS-Simulink Converter14/1 -> Scope4/1, If3/1
  Constant6/1 -> If Action Subsystem6/1(In1)
  Constant7/1 -> If Action Subsystem7/1(In1)
  PS-Simulink Converter15/1 -> If5/1, Scope5/1
  If Action Subsystem7/1(Out1) -> Simulink-PS Converter12/1
  If5/1 -> If Action Subsystem7/Action
  connections:
  Inside Edge SA1/LConn1 -- Top SA1/RConn1 -- SA1/LConn1
  SA2/LConn1 -- Outside Edge SA2/RConn1 -- Top SA2/RConn1
  Hinge 1 to SA1/RConn1 -- Hinge 1/LConn1 -- Hinge 1 to +X Chassis/LConn1
  Hinge 2/LConn1 -- Hinge 2 to +X Chassis/RConn1 -- Hinge 2 to SA2/LConn1
  +X Chassis to Hinge 2/LConn1 -- +X Chassis/LConn1 -- Temperature Sensor3/LConn1 -- "Bottom +X Chassis "/LConn1 -- "Top +X Chassis "/RConn1 -- +X Chassis to Hinge 1/RConn1
  Top -X Chassis/RConn1 -- -X Chassis to Outside/RConn1 -- -X Chassis to XRD/LConn1 -- -X Chassis to GRD/LConn1 -- Temperature Sensor6/LConn1 -- +X Chassis1/LConn1
  Top +Z Chassis/RConn1 -- +Z Chassis to Radiator/RConn1 -- +Z Chassis to Outside/RConn1 -- +Z Chassis to XRD/LConn1 -- +Z Chassis to GRD/LConn1 -- +Z Chassis to +Y Chassis/RConn1 -- Temperature Sensor2/LConn1 -- +Z Chassis to -X Chassis/LConn1 -- +Z Chassis/LConn1 -- +Z Chassis to -Y Chassis/LConn1 -- +Z Chassis to Inside/LConn1
  +Y Chassis/LConn1 -- +Y Chassis to -Z Chassis/LConn1 -- Temperature Sensor10/LConn1 -- +Y Chassis to -X Chassis/LConn1 -- +Y Chassis to GRD/LConn1 -- +Y Chassis to XRD/LConn1 -- Top +Y Chassis/RConn1 -- +Y Chassis to Outside/LConn1 -- +Y Chassis to Inside/RConn1 -- +Y Chassis to +Z Chassis/RConn1
  "Top -Y Chassis "/RConn1 -- -Y to Outside/LConn1 -- -Y to Inside/RConn1 -- Temperature Sensor8/LConn1 -- "Bottom -Y Chassis "/LConn1 -- -Y Chassis/LConn1 -- -Y Chassis to +Z Chassis/LConn1 -- -Y Chassis to -Z Chassis/RConn1
  Inside Edge SA1/RConn1 -- Hinge 1 to SA1/LConn1
  Hinge 1 to +X Chassis/RConn1 -- +X Chassis to Hinge 1/LConn1
  +X Chassis to Hinge 2/RConn1 -- Hinge 2 to +X Chassis/LConn1
  Hinge 2 to SA2/RConn1 -- Outside Edge SA2/LConn1
  "Bottom +X Chassis "/RConn1 -- "Top -Y Chassis "/LConn1 -- Top +Y Chassis/LConn1 -- Top +Z Chassis/LConn1
  +Z Chassis to -Y Chassis/RConn1 -- +Y Chassis to +Z Chassis/LConn1
  +Z Radiator to +Z Chassis/RConn1 -- +Z Chassis to Radiator/LConn1
  +Z Radiator to Space/RConn1 -- +Z Radiator/LConn1 -- +Z Radiator to +Z Chassis/LConn1
  +Z Chassis to +Y Chassis/LConn1 -- Top -Z Chassis/LConn1 -- -Y Chassis to +Z Chassis/RConn1
  -Z Chassis/LConn1 -- Controlled Heat Flow Rate Source11/LConn1 -- Temperature Sensor14/LConn1 -- -Z Chassis to GRD/LConn1 -- -Z Chassis to XRD/LConn1 -- -Z Chassis to Outside/RConn1 -- -Z Chassis to Radiator/RConn1 -- Top -Z Chassis/RConn1 -- -Z Chassis to Inside/LConn1 -- Temperature Sensor9/LConn1 -- -Z Chassis to -X Chassis1/LConn1 -- -Z Chassis to -Y Chassis/RConn1 -- -Z Chassis to +Y Chassis/LConn1
  -Z Radiator/LConn1 -- -Z Radiator to -Z Chassis/LConn1 -- -Z Radiator to Space/RConn1
  -Z Radiator to -Z Chassis/RConn1 -- -Z Chassis to Radiator/LConn1
  -Z Chassis to +Y Chassis/RConn1 -- -Y Chassis to -Z Chassis/LConn1
  -Z Chassis to -Y Chassis/LConn1 -- +Y Chassis to -Z Chassis/RConn1
  Radiative Heat Transfer/LConn1 -- Controlled Heat Flow Rate Source/LConn1 -- +Z Chassis to Outside/LConn1
  Simulink-PS Converter/RConn1 -- Controlled Heat Flow Rate Source/RConn1
  Thermal Reference/LConn1 -- Controlled Heat Flow Rate Source/RConn2
  Heat Flow Rate Sensor4/RConn2 -- Space/LConn1
  +Z Chassis to -X Chassis/RConn1 -- +Y Chassis to -X Chassis/RConn1 -- "Bottom -Y Chassis "/RConn1 -- -Z Chassis to -X Chassis1/RConn1 -- Top -X Chassis/LConn1
  Controlled Heat Flow Rate Source1/LConn1 -- -Z Chassis to Outside/LConn1 -- Radiative Heat Transfer1/LConn1
  Thermal Reference1/LConn1 -- Controlled Heat Flow Rate Source1/RConn2
  Simulink-PS Converter1/RConn1 -- Controlled Heat Flow Rate Source1/RConn1
  Heat Flow Rate Sensor7/RConn2 -- Space1/LConn1
  Thermal Reference2/LConn1 -- Controlled Heat Flow Rate Source2/RConn2
  Simulink-PS Converter2/RConn1 -- Controlled Heat Flow Rate Source2/RConn1
  Heat Flow Rate Sensor5/RConn2 -- Space2/LConn1
  Controlled Heat Flow Rate Source2/LConn1 -- Radiative Heat Transfer2/LConn1 -- -X Chassis to Outside/LConn1
  +Z Chassis to Inside/RConn1 -- Avionics Box to +Y/RConn1 -- +Y Chassis to Inside/LConn1 -- Avionics Box to +Z/LConn1
  Avionics Box to +Z/RConn1 -- Temperature Sensor13/LConn1 -- Temperature Sensor15/LConn1 -- Avionics Box/LConn1 -- Controlled Heat Flow Rate Source10/LConn1 -- Avionics Bottom/LConn1 -- Avionics Top/RConn1 -- Avionics Box to +Y/LConn1 -- Avionics -Y/LConn1 -- Avionics -Z/RConn1 -- Controlled Heat Flow Rate Source12/LConn1 -- Temperature Sensor5/LConn1
  Avionics -Y/RConn1 -- Battery Box to Avionics/LConn1
  Battery Box to Avionics/RConn1 -- Temperature Sensor12/LConn1 -- Controlled Heat Flow Rate Source8/LConn1 -- Temperature Sensor4/LConn1 -- Battery Box/LConn1 -- Thermal Resistance/RConn1 -- Controlled Heat Flow Rate Source9/LConn1
  +Z GRD/LConn1 -- +Z Chassis to GRD/RConn1
  +Z XRD/LConn1 -- +Z Chassis to XRD/RConn1
  +Y XRD/LConn1 -- +Y Chassis to XRD/RConn1
  +Y GRD/LConn1 -- +Y Chassis to GRD/RConn1
  -Z GRD/LConn1 -- -Z Chassis to GRD/RConn1
  -Z XRD/LConn1 -- -Z Chassis to XRD/RConn1
  -X XRD/LConn1 -- Temperature Sensor11/LConn1 -- -X Chassis to XRD/RConn1
  -X GRD/LConn1 -- -X Chassis to GRD/RConn1
  Space3/LConn1 -- Heat Flow Rate Sensor3/RConn2
  Radiative Heat Transfer3/LConn1 -- +Z Radiator to Space/LConn1
  Radiative Heat Transfer4/LConn1 -- Controlled Heat Flow Rate Source3/LConn1 -- +Y Chassis to Outside/RConn1
  Heat Flow Rate Sensor8/RConn2 -- Space4/LConn1
  Thermal Reference3/LConn1 -- Controlled Heat Flow Rate Source3/RConn2
  Simulink-PS Converter3/RConn1 -- Controlled Heat Flow Rate Source3/RConn1
  Heat Flow Rate Sensor6/RConn2 -- Space5/LConn1
  -Z Radiator to Space/LConn1 -- Radiative Heat Transfer5/LConn1
  -Z Chassis to Inside/RConn1 -- Perfect Insulator/LConn1
  Perfect Insulator1/LConn1 -- -Y to Inside/LConn1
  Controlled Heat Flow Rate Source4/LConn1 -- Radiative Heat Transfer6/LConn1 -- -Y to Outside/RConn1
  Simulink-PS Converter4/RConn1 -- Controlled Heat Flow Rate Source4/RConn1
  Heat Flow Rate Sensor9/RConn2 -- Space6/LConn1
  Thermal Reference4/LConn1 -- Controlled Heat Flow Rate Source4/RConn2
  Radiative Heat Transfer7/LConn1 -- Controlled Heat Flow Rate Source5/LConn1 -- Temperature Sensor1/LConn1 -- Top SA1/LConn1
  Heat Flow Rate Sensor2/LConn1 -- Radiative Heat Transfer7/RConn1
  Thermal Reference5/LConn1 -- Controlled Heat Flow Rate Source5/RConn2
  Simulink-PS Converter5/RConn1 -- Controlled Heat Flow Rate Source5/RConn1
  Controlled Heat Flow Rate Source6/LConn1 -- Radiative Heat Transfer8/LConn1 -- "Top +X Chassis "/LConn1
  Simulink-PS Converter6/RConn1 -- Controlled Heat Flow Rate Source6/RConn1
  Thermal Reference6/LConn1 -- Controlled Heat Flow Rate Source6/RConn2
  Heat Flow Rate Sensor1/RConn2 -- Space8/LConn1
  Controlled Heat Flow Rate Source7/LConn1 -- Radiative Heat Transfer9/LConn1 -- Top SA2/LConn1
  Simulink-PS Converter7/RConn1 -- Controlled Heat Flow Rate Source7/RConn1
  Thermal Reference7/LConn1 -- Controlled Heat Flow Rate Source7/RConn2
  Solver Configuration/RConn1 -- Temperature Sensor7/LConn1 -- Thermal Resistance/LConn1
  Temperature Sensor1/RConn2 -- Solar Array/LConn1
  Thermal Reference8/LConn1 -- Temperature Sensor1/RConn1
  Thermal Reference9/LConn1 -- Temperature Sensor3/RConn1
  Thermal Reference12/LConn1 -- Temperature Sensor4/RConn1
  Temperature Sensor4/RConn2 -- BatteryBox/LConn1
  Thermal Reference13/LConn1 -- Temperature Sensor5/RConn1
  Temperature Sensor5/RConn2 -- AvionicsBox/LConn1
  Thermal Reference14/LConn1 -- Temperature Sensor6/RConn1
  Temperature Sensor6/RConn2 -- X- chassis face/LConn1
  Heat Flow Rate Sensor1/RConn1 -- PS-Simulink Converter2/LConn1
  PS-Simulink Converter3/LConn1 -- Heat Flow Rate Sensor10/RConn1
  Heat Flow Rate Sensor3/RConn1 -- PS-Simulink Converter4/LConn1
  Heat Flow Rate Sensor4/RConn1 -- PS-Simulink Converter5/LConn1
  Heat Flow Rate Sensor5/RConn1 -- PS-Simulink Converter6/LConn1
  Heat Flow Rate Sensor6/RConn1 -- PS-Simulink Converter7/LConn1
  Heat Flow Rate Sensor7/RConn1 -- PS-Simulink Converter8/LConn1
  Heat Flow Rate Sensor8/RConn1 -- PS-Simulink Converter9/LConn1
  Heat Flow Rate Sensor9/RConn1 -- PS-Simulink Converter10/LConn1
  Thermal Reference16/LConn1 -- Controlled Heat Flow Rate Source8/RConn2
  Simulink-PS Converter9/RConn1 -- Controlled Heat Flow Rate Source8/RConn1
  PS-Simulink Converter11/LConn1 -- Temperature Sensor7/RConn2
  Thermal Reference15/LConn1 -- Temperature Sensor7/RConn1
  PS-Simulink Converter12/LConn1 -- Heat Flow Rate Sensor2/RConn1
  Space7/LConn1 -- Heat Flow Rate Sensor2/RConn2
  Heat Flow Rate Sensor1/LConn1 -- Radiative Heat Transfer8/RConn1
  Heat Flow Rate Sensor10/RConn2 -- Space9/LConn1
  Heat Flow Rate Sensor10/LConn1 -- Radiative Heat Transfer9/RConn1
  Heat Flow Rate Sensor9/LConn1 -- Radiative Heat Transfer6/RConn1
  Heat Flow Rate Sensor5/LConn1 -- Radiative Heat Transfer2/RConn1
  Heat Flow Rate Sensor8/LConn1 -- Radiative Heat Transfer4/RConn1
  Heat Flow Rate Sensor6/LConn1 -- Radiative Heat Transfer5/RConn1
  Heat Flow Rate Sensor7/LConn1 -- Radiative Heat Transfer1/RConn1
  Heat Flow Rate Sensor3/LConn1 -- Radiative Heat Transfer3/RConn1
  Heat Flow Rate Sensor4/LConn1 -- Radiative Heat Transfer/RConn1
  Controlled Heat Flow Rate Source9/RConn2 -- Thermal Reference10/LConn1
  Simulink-PS Converter8/RConn1 -- Controlled Heat Flow Rate Source9/RConn1
  Simulink-PS Converter10/RConn1 -- Controlled Heat Flow Rate Source10/RConn1
  Controlled Heat Flow Rate Source10/RConn2 -- Thermal Reference11/LConn1
  Thermal Reference17/LConn1 -- Temperature Sensor2/RConn1
  Temperature Sensor2/RConn2 -- Z+ chassis Face/LConn1
  Temperature Sensor3/RConn2 -- X+ chassis face/LConn1
  Temperature Sensor9/RConn1 -- Thermal Reference19/LConn1
  Temperature Sensor9/RConn2 -- Z- chassis face/LConn1
  Temperature Sensor8/RConn1 -- Thermal Reference18/LConn1
  Temperature Sensor8/RConn2 -- Y- chassis face/LConn1
  Temperature Sensor10/RConn1 -- Thermal Reference20/LConn1
  Temperature Sensor10/RConn2 -- Y+ chassis face/LConn1
  Temperature Sensor11/RConn1 -- Thermal Reference21/LConn1
  Temperature Sensor11/RConn2 -- XRD (X-)/LConn1
  Thermal Reference22/LConn1 -- Temperature Sensor12/RConn1
  Temperature Sensor12/RConn2 -- PS-Simulink Converter1/LConn1
  Temperature Sensor13/RConn2 -- PS-Simulink Converter13/LConn1
  Thermal Reference23/LConn1 -- Temperature Sensor13/RConn1
  PS-Simulink Converter14/LConn1 -- Temperature Sensor14/RConn2
  Thermal Reference25/LConn1 -- Controlled Heat Flow Rate Source11/RConn2
  Simulink-PS Converter11/RConn1 -- Controlled Heat Flow Rate Source11/RConn1
  Thermal Reference24/LConn1 -- Temperature Sensor14/RConn1
  Simulink-PS Converter12/RConn1 -- Controlled Heat Flow Rate Source12/RConn1
  Thermal Reference27/LConn1 -- Controlled Heat Flow Rate Source12/RConn2
  PS-Simulink Converter15/LConn1 -- Temperature Sensor15/RConn2
  Thermal Reference26/LConn1 -- Temperature Sensor15/RConn1
